simulink model "one_step"  (R2024a)
settings: Solver=ode45  StartTime=0.0  StopTime=ttt  MaxStep=0.0001  RelTol=1e-4  AbsTol=1e-4
values from neighbouring files (symbols this model uses):
  dt = 0.01    [OneStepSim.m]
settings Model: Creator=stanl  LastModifiedBy=stanl

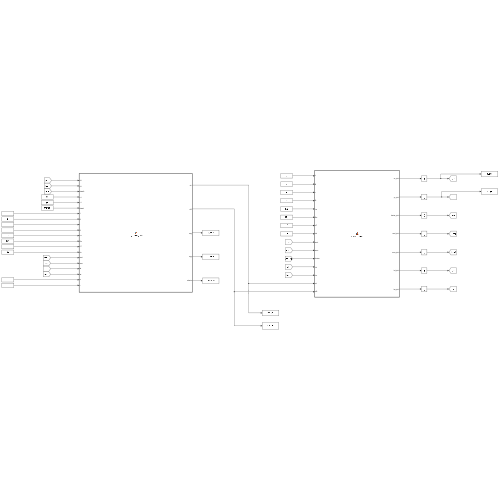
[thumbnail: Simulink's stored preview of the top-level diagram]
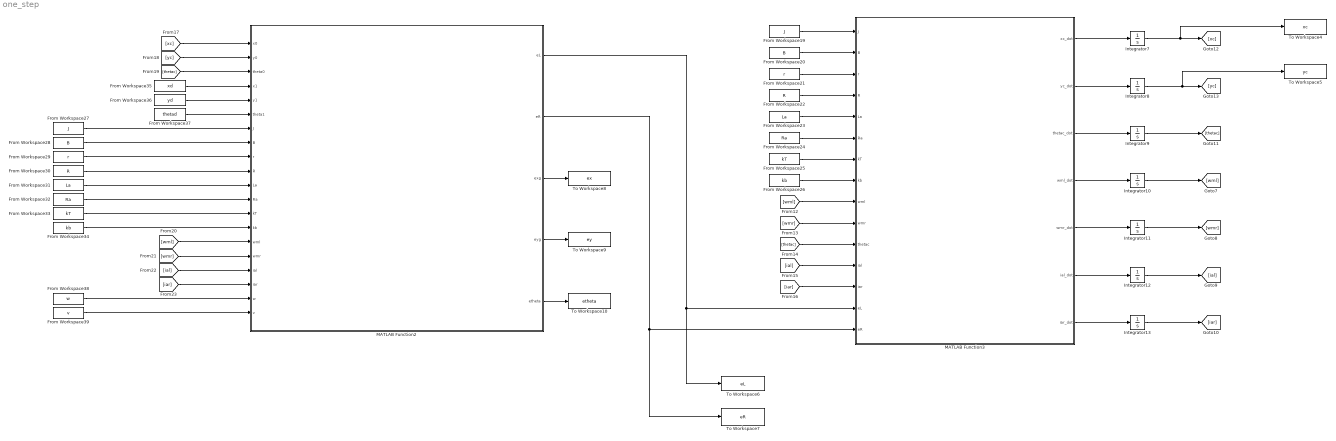
== system one_step ==
  From Workspace19 : FromWorkspace  VariableName=J  SampleTime=dt
  From Workspace20 : FromWorkspace  VariableName=B  SampleTime=dt
  From Workspace21 : FromWorkspace  VariableName=r  SampleTime=dt
  From Workspace22 : FromWorkspace  VariableName=R  SampleTime=dt
  From Workspace23 : FromWorkspace  VariableName=La  SampleTime=dt
  From Workspace24 : FromWorkspace  VariableName=Ra  SampleTime=dt
  From Workspace25 : FromWorkspace  VariableName=kT  SampleTime=dt
  From Workspace26 : FromWorkspace  VariableName=kb  SampleTime=dt
  From Workspace27 : FromWorkspace  VariableName=J  SampleTime=dt
  From Workspace28 : FromWorkspace  VariableName=B  SampleTime=dt
  From Workspace29 : FromWorkspace  VariableName=r  SampleTime=dt
  From Workspace30 : FromWorkspace  VariableName=R  SampleTime=dt
  From Workspace31 : FromWorkspace  VariableName=La  SampleTime=dt
  From Workspace32 : FromWorkspace  VariableName=Ra  SampleTime=dt
  From Workspace33 : FromWorkspace  VariableName=kT  SampleTime=dt
  From Workspace34 : FromWorkspace  VariableName=kb  SampleTime=dt
  From Workspace35 : FromWorkspace  VariableName=xd  SampleTime=dt
  From Workspace36 : FromWorkspace  VariableName=yd  SampleTime=dt
  From Workspace37 : FromWorkspace  VariableName=thetad  SampleTime=dt
  From Workspace38 : FromWorkspace  VariableName=w  SampleTime=dt
  From Workspace39 : FromWorkspace  VariableName=v  SampleTime=dt
  Integrator{8..13} (6 alike) : Integrator
  Integrator7 : Integrator  InitialCondition=-1
  MATLAB Function2 : MATLAB Function  TreatAsAtomicUnit=on  SystemSampleTime=dt
  MATLAB Function3 : MATLAB Function  TreatAsAtomicUnit=on  SystemSampleTime=dt
  To Workspace10 : ToWorkspace  VariableName=etheta  SaveFormat=Timeseries  SampleTime=dt
  To Workspace4 : ToWorkspace  VariableName=xc  SaveFormat=Timeseries  SampleTime=dt
  To Workspace5 : ToWorkspace  VariableName=yc  SaveFormat=Timeseries  SampleTime=dt
  To Workspace6 : ToWorkspace  VariableName=eL  SaveFormat=Timeseries  SampleTime=dt
  To Workspace7 : ToWorkspace  VariableName=eR  SaveFormat=Timeseries  SampleTime=dt
  To Workspace8 : ToWorkspace  VariableName=ex  SaveFormat=Timeseries  SampleTime=dt
  To Workspace9 : ToWorkspace  VariableName=ey  SaveFormat=Timeseries  SampleTime=dt
  wires:
  MATLAB Function3/1(xc_dot) -> Integrator7/1
  Integrator7/1 -> To Workspace4/1, [xc]
  [wmr] -> MATLAB Function3/10(wmr)
  From Workspace26/1 -> MATLAB Function3/8(kb)
  [ial] -> MATLAB Function3/12(ial)
  Integrator11/1 -> [wmr]
  Integrator12/1 -> [ial]
  From Workspace22/1 -> MATLAB Function3/4(R)
  From Workspace19/1 -> MATLAB Function3/1(J)
  Integrator8/1 -> To Workspace5/1, [yc]
  MATLAB Function3/6(ial_dot) -> Integrator12/1
  From Workspace25/1 -> MATLAB Function3/7(kT)
  MATLAB Function2/2(eR) -> To Workspace7/1, MATLAB Function3/15(eR)
  [wml] -> MATLAB Function3/9(wml)
  [thetac] -> MATLAB Function3/11(thetac)
  Integrator9/1 -> [thetac]
  From Workspace24/1 -> MATLAB Function3/6(Ra)
  From Workspace23/1 -> MATLAB Function3/5(La)
  From Workspace20/1 -> MATLAB Function3/2(B)
  Integrator13/1 -> [iar]
  MATLAB Function3/2(yc_dot) -> Integrator8/1
  [iar] -> MATLAB Function3/13(iar)
  MATLAB Function3/3(thetac_dot) -> Integrator9/1
  MATLAB Function3/5(wmr_dot) -> Integrator11/1
  MATLAB Function2/1(eL) -> To Workspace6/1, MATLAB Function3/14(eL)
  Integrator10/1 -> [wml]
  MATLAB Function3/4(wml_dot) -> Integrator10/1
  MATLAB Function3/7(iar_dot) -> Integrator13/1
  From Workspace21/1 -> MATLAB Function3/3(r)
  From Workspace27/1 -> MATLAB Function2/7(J)
  From Workspace28/1 -> MATLAB Function2/8(B)
  From Workspace29/1 -> MATLAB Function2/9(r)
  From Workspace30/1 -> MATLAB Function2/10(R)
  From Workspace31/1 -> MATLAB Function2/11(La)
  From Workspace32/1 -> MATLAB Function2/12(Ra)
  From Workspace33/1 -> MATLAB Function2/13(kT)
  From Workspace34/1 -> MATLAB Function2/14(kb)
  From Workspace35/1 -> MATLAB Function2/4(x1)
  From Workspace36/1 -> MATLAB Function2/5(y1)
  From Workspace37/1 -> MATLAB Function2/6(theta1)
  [xc] -> MATLAB Function2/1(x0)
  [yc] -> MATLAB Function2/2(y0)
  [thetac] -> MATLAB Function2/3(theta0)
  [wml] -> MATLAB Function2/15(wml)
  [wmr] -> MATLAB Function2/16(wmr)
  [ial] -> MATLAB Function2/17(ial)
  [iar] -> MATLAB Function2/18(iar)
  MATLAB Function2/3(exg) -> To Workspace8/1
  MATLAB Function2/4(eyg) -> To Workspace9/1
  MATLAB Function2/5(etheta) -> To Workspace10/1
  From Workspace38/1 -> MATLAB Function2/19(w)
  From Workspace39/1 -> MATLAB Function2/20(v)

== matlab function one_step/MATLAB Function2 ==
  data: x0 input; eL output; eR output; y0 input; theta0 input; x1 input; y1 input; theta1 input; J input; B input; r input; R input; La input; Ra input; kT input; kb input; wml input; wmr input; ial input; iar input; exg output; eyg output; etheta output; w input; v input
function [eL,eR,exg,eyg,etheta] = first_control_block(x0,y0,theta0,x1,y1,theta1,J,B,r,R,La,Ra,kT,kb,wml,wmr,ial,iar,w,v)
persistent xd_pre yd_pre theta_pre xdot_f ydot_f wd_f initialized wml_ref_pre wmr_ref_pre
t=0.01;
if isempty(initialized)
    xd_pre=x1;
    yd_pre=y1;
    theta_pre=theta1;
    xdot_f=0;
    ydot_f=0;
    wd_f=0;
    initialized=true;
    wml_ref_pre=0;
    wmr_ref_pre=0;
end
dt=t;
tau_v=0.05;
alpha_v=dt/(tau_v+dt);
xdot=(x1-xd_pre)/dt;
ydot=(y1-yd_pre)/dt;
xdot_f=(1-alpha_v)*xdot_f+alpha_v*xdot;
ydot_f=(1-alpha_v)*ydot_f+alpha_v*ydot;
vdd=sqrt(xdot_f*xdot_f+ydot_f*ydot_f);
if(vdd<1e-6)
    theta_inst=theta_pre;
else
    theta_inst=atan2(ydot_f,xdot_f);
end
dtheta=atan2(sin(theta_inst-theta_pre),cos(theta_inst-theta_pre));
theta_d=theta_pre+dtheta;

tau_w=0.05;
alpha_w=dt/(tau_w+dt);
wd_raw=dtheta/dt;
wd_f=(1-alpha_w)*wd_f+alpha_w*wd_raw;
wdd=wd_f;

xd_pre=x1;
yd_pre=y1;
theta_pre=theta1;

T=[cos(theta0) sin(theta0) 0;
    -sin(theta0) cos(theta0) 0;
    0 0 1];
theta_error=atan2(sin(theta0-theta1),cos(theta0-theta1));
Pe=T*[x0-x1;y0-y1;theta_error];
ex=Pe(1);
ey=Pe(2);
etheta=Pe(3);

exg=x0-x1;
eyg=y0-y1;
ethetag=theta_error;

vdd=v;
wdd=w;

kv=10.0048; kw=1.9952; ky=11.5606;
vc=-kv*ex+vdd*cos(etheta);
wc=wdd-ky*ey*vdd-kw*sin(etheta);
% vc=kv*ex+vdd*cos(etheta);
% wc=wdd+ky*ey*vdd+kw*sin(etheta);

vcmax=2;
wcmax=3;
vc=max(-vcmax,min(vcmax,vc));
wc=max(-wcmax,min(wcmax,wc));

% vc=-kv*ex+vdd*cos(etheta)+(-1+kw)*ey*vdd*sin(etheta);
% wc=wdd-kw*ey*vdd-kw*sin(etheta);
wmR_ref=(1/r)*(vc+R*wc);
wmL_ref=(1/r)*(vc-R*wc);
wmL_ref=min(max(wmL_ref,-22.24),22.24);
wmR_ref=min(max(wmR_ref,-22.24),22.24);

% A=[-B/J kT/J;
%    -kb/La -Ra/La];
% B=[0;1/La];
% C=[1 0];
% 
% eL=( wmL_ref-C*expm(A*t)*[wml;ial] )/( C*inv(A)*(expm(A*t)-eye(2))*B );
% eR=( wmR_ref-C*expm(A*t)*[wmr;iar] )/( C*inv(A)*(expm(A*t)-eye(2))*B );

a=(Ra*J)/kT;
b=(Ra*B)/kT + kb;
eL=a*(wmL_ref-wml_ref_pre)/dt + b*wmL_ref;
eR=a*(wmR_ref-wmr_ref_pre)/dt + b*wmR_ref;
wml_ref_pre=wmL_ref;
wmr_ref_pre=wmR_ref;


% if( abs(Dtheta)>1e-6 )
%     omega=Dtheta/t;
%     denx=sin(theta0+Dtheta)-sin(theta0);
%     deny=-cos(theta0+Dtheta)+cos(theta0);
%     vx=(Dx*omega)/max(denx,1e-12*sign(denx));
%     vy=(Dy*omega)/max(deny,1e-12*sign(deny));
%     v=0.5*(vx+vy);
% else
%     omega=0;
%     v=(Dx*cos(theta0)+Dy*sin(theta0))/t;
% end
% wml_ref=(v-R*omega)/r;
% wmr_ref=(v+R*omega)/r;
% 
% A=[-B/J kT/J;
%    -kb/La -Ra/La];
% B=[0;1/La];
% C=[1 0];
% phi=expm(A*t);
% gamma=(A\(phi-eye(2)))*B;
% 
% % eL=(wml_ref - C*(phi*[wml;ial]))/(C*gamma);
% % eR=(wmr_ref - C*(phi*[wmr;iar]))/(C*gamma);
% 
% G1    = (A \ (phi - eye(2)));                    % A^{-1}(Phi-I)
% G2    = (A \ (G1 - t*eye(2))) * B;              % A^{-1}( A^{-1}(Phi-I) - tI ) * B
% bias  = C * (G1 * [wml;ial]);                    % 對應 x0 的項
% % 目標平均輪速 = 反解得到的 wm*_ref
% eL = ( wml_ref * t - bias ) / ( C * G2 );
% % 右輪
% bias = C * (G1 * [wmr;iar]);
% eR = ( wmr_ref * t - bias ) / ( C * G2 );

eL=min(max(eL,-12),12);
eR=min(max(eR,-12),12);

end

== matlab function one_step/MATLAB Function3 ==
  data: J input; B input; r input; R input; La input; Ra input; kT input; kb input; wml input; wmr input; thetac input; ial input; iar input; eL input; eR input; xc_dot output; yc_dot output; thetac_dot output; wml_dot output; wmr_dot output; ial_dot output; iar_dot output
function [xc_dot,yc_dot,thetac_dot,wml_dot,wmr_dot,ial_dot,iar_dot]=vehcile_system(J,B,r,R,La,Ra,kT,kb,wml,wmr,thetac,ial,iar,eL,eR)

xc_dot=0.5*r*(wml+wmr)*cos(thetac);
yc_dot=0.5*r*(wml+wmr)*sin(thetac);
thetac_dot=(r/(2*R))*(wmr-wml);
wml_dot=(-B/J)*wml+(kT/J)*ial;
wmr_dot=(-B/J)*wmr+(kT/J)*iar;
ial_dot=(-kb/La)*wml-(Ra/La)*ial+(1/La)*eL;
iar_dot=(-kb/La)*wmr-(Ra/La)*iar+(1/La)*eR;

% xc_dot=0.5*r*(wml+wmr)*cos(thetac);
% yc_dot=0.5*r*(wml+wmr)*sin(thetac);
% thetac_dot=(r/(2*R))*(wmr-wml);
% wml_dot=-(B/J + (kb*kT)/(Ra*J))*wml+(kT/(Ra*J))*eL;
% wmr_dot=-(B/J + (kb*kT)/(Ra*J))*wmr+(kT/(Ra*J))*eR;
% ial_dot=0;
% iar_dot=0;
end
